simulink model "DiscreteIntegrator_TestGen14"  (R2017b)
settings: Solver=FixedStepDiscrete  StartTime=0.0  StopTime=10.0  RelTol=1e-3
undefined symbols (not defined in the file): DiscIntNeverNeededParam
settings Model: Creator=hbourbou  LastModifiedBy=hbourbou
settings DebuggingCC: ParameterOverflowMsg=none

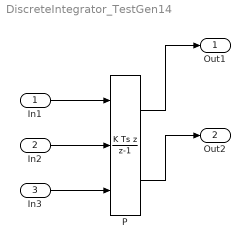
== system DiscreteIntegrator_TestGen14 ==
  In1 : Inport  OutDataTypeStr=uint8  PortDimensions=[2,3]
  In2 : Inport  Port=2
  In3 : Inport  Port=3
  P : DiscreteIntegrator  IntegratorMethod=Integration: Backward Euler  gainval=2.0  ExternalReset=either  InitialConditionSource=external  InitialCondition=7  SampleTime=-1  OutDataTypeStr=uint8  RndMeth=Zero  SaturateOnIntegerOverflow=on  LimitOutput=on  UpperSaturationLimit=100  LowerSaturationLimit=5  ShowSaturationPort=on  ShowStatePort=on  ICPrevOutput=DiscIntNeverNeededParam  ICPrevScaledInput=DiscIntNeverNeededParam
  Out1 : Outport
  Out2 : Outport  Port=2
  wires:
  In1/1 -> P/1
  In2/1 -> P/2
  In3/1 -> P/3
  P/1 -> Out1/1
  P/2 -> Out2/1
